simulink model "part1"  (R2021b)
settings: Solver=VariableStepAuto  StartTime=0.0  StopTime=10  RelTol=1e-3
settings Model: Creator=chand  LastModifiedBy=chand

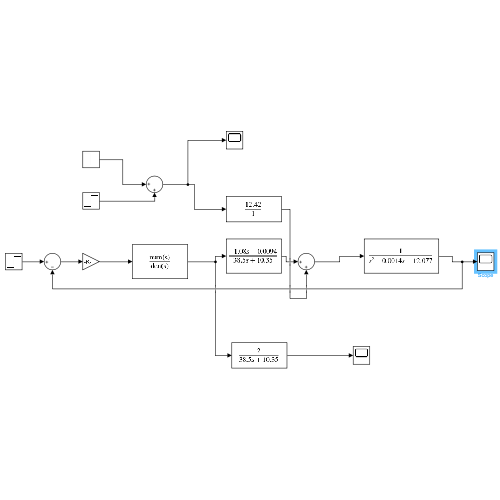
[thumbnail: Simulink's stored preview of the top-level diagram]
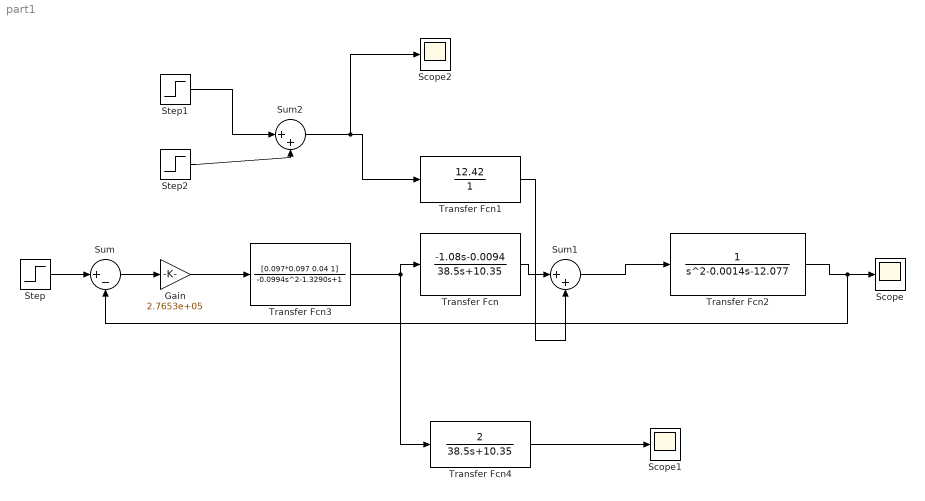
== system part1 ==
  Gain : Gain  Gain=2.7653e+05
  Scope : Scope
  Scope1 : Scope
  Scope2 : Scope
  Step : Step  After=0  SampleTime=0
  Step1 : Step  After=-1  SampleTime=0
  Step2 : Step  Time=0  SampleTime=0
  Sum : Sum  Inputs=|+-
  Sum1 : Sum  Inputs=|++
  Sum2 : Sum  Inputs=|++
  Transfer Fcn : TransferFcn  Numerator=[-1.08 -0.0094]  Denominator=[38.5 10.35]
  Transfer Fcn1 : TransferFcn  Numerator=[12.42]  Denominator=[1]
  Transfer Fcn2 : TransferFcn  Denominator=[1 -0.0014 -12.077]
  Transfer Fcn3 : TransferFcn  Numerator=[0.097*0.097 0.04 1]  Denominator=[-0.0994 -1.3290 1]
  Transfer Fcn4 : TransferFcn  Numerator=[2]  Denominator=[38.5 10.35]
  wires:
  Transfer Fcn/1 -> Sum1/1
  Transfer Fcn2/1 -> Sum/2, Scope/1
  Transfer Fcn4/1 -> Scope1/1
  Sum1/1 -> Transfer Fcn2/1
  Transfer Fcn1/1 -> Sum1/2
  Transfer Fcn3/1 -> Transfer Fcn4/1, Transfer Fcn/1
  Step/1 -> Sum/1
  Sum/1 -> Gain/1
  Gain/1 -> Transfer Fcn3/1
  Step2/1 -> Sum2/2
  Step1/1 -> Sum2/1
  Sum2/1 -> Scope2/1, Transfer Fcn1/1
